simulink model "stepper_motor"  (R2015b)
settings: Solver=FixedStepDiscrete  StartTime=0.0  StopTime=0.25  FixedStep=Ts  RelTol=1e-3
undefined symbols (not defined in the file): DiscIntNeverNeededParam, Ts
settings Model: Creator=YogurtSuee  LastModifiedBy=YogurtSuee

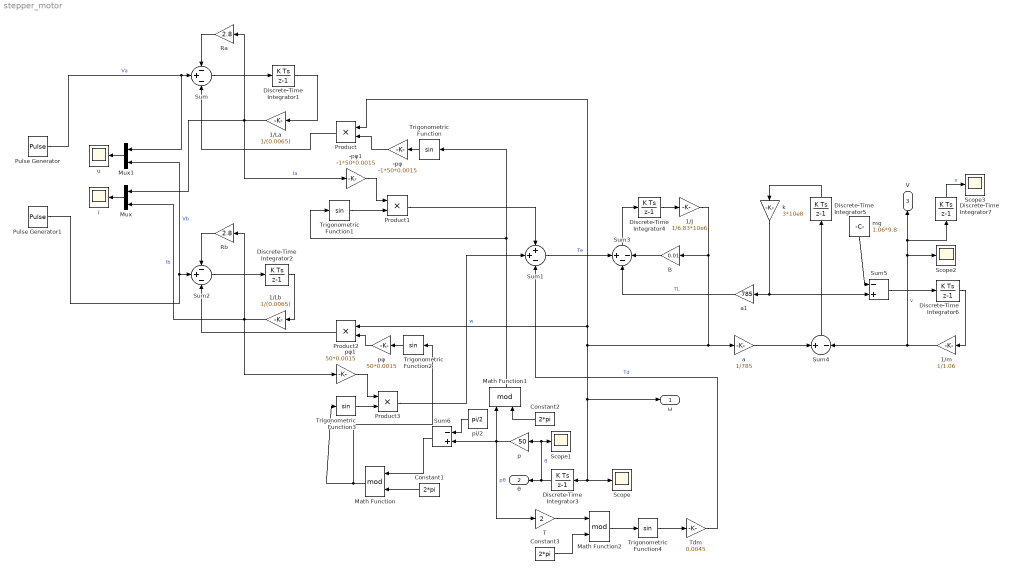
== system stepper_motor ==
  -pφ : Gain  Gain=-1*50*0.0015
  -pφ1 : Gain  Gain=-1*50*0.0015
  1/J : Gain  Gain=1/6.83*10e6
  1/La : Gain  Gain=1/(0.0065)
  1/Lb : Gain  Gain=1/(0.0065)
  1/m : Gain  Gain=1/1.06
  B : Gain  Gain=0.01
  Constant1 : Constant  Value=2*pi
  Constant2 : Constant  Value=2*pi
  Constant3 : Constant  Value=2*pi
  Discrete-Time Integrator{1..7} (7 alike) : DiscreteIntegrator  SampleTime=Ts  ICPrevOutput=DiscIntNeverNeededParam  ICPrevScaledInput=DiscIntNeverNeededParam
  Math Function : Math  Operator=mod  SaturateOnIntegerOverflow=on
  Math Function1 : Math  Operator=mod  SaturateOnIntegerOverflow=on
  Math Function2 : Math  Operator=mod  SaturateOnIntegerOverflow=on
  Mux : Mux  Inputs=2
  Mux1 : Mux  Inputs=2
  Product{,1..3} (4 alike) : Product
  Pulse Generator : DiscretePulseGenerator  PulseType=Time based  Amplitude=24  Period=0.02  PulseWidth=10  SampleTime=0.2
  Pulse Generator1 : DiscretePulseGenerator  PulseType=Time based  Amplitude=24  Period=0.02  PulseWidth=10  PhaseDelay=0.01  SampleTime=0.2
  Ra : Gain  Gain=2.8
  Rb : Gain  Gain=2.8
  Scope{,1..3} (4 alike) : Scope
  Sum : Sum  Inputs=-+-
  Sum1 : Sum  Inputs=++-
  Sum2 : Sum  Inputs=-+-
  Sum3 : Sum  Inputs=+--
  Sum4 : Sum  Inputs=+-
  Sum5 : Sum  Inputs=-+
  Sum6 : Sum  Inputs=-+
  T : Gain  Gain=2
  Tdm : Gain  Gain=0.0045
  Trigonometric Function{,1..2,4} (4 alike) : Trigonometry
  Trigonometric Function3 : Trigonometry  OutputSignalType=real
  a : Gain  Gain=1/785
  a1 : Gain  Gain=785
  i : Scope
  k : Gain  Gain=3*10e8
  mg : Constant  Value=1.06*9.8
  p : Gain  Gain=50
  pi/2 : Constant  Value=pi/2
  pφ : Gain  Gain=50*0.0015
  pφ1 : Gain  Gain=50*0.0015
  u : Scope
  ω : Outport
  θ : Outport  Port=2
  V : Outport  Port=3
  wires:
  Discrete-Time Integrator1/1 -> 1/La/1
  Sum/1 -> Discrete-Time Integrator1/1
  Ra/1 -> Sum/1
  1/La/1 -> -pφ1/1, Mux/1, Ra/1  "Ia"
  Product/1 -> Sum/3
  -pφ1/1 -> Product1/1
  Trigonometric Function1/1 -> Product1/2
  Product1/1 -> Sum1/1
  Discrete-Time Integrator2/1 -> 1/Lb/1
  Sum2/1 -> Discrete-Time Integrator2/1
  Rb/1 -> Sum2/1
  1/Lb/1 -> pφ1/1, Mux/2, Rb/1  "Ib"
  Product2/1 -> Sum2/3
  pφ1/1 -> Product3/1
  Trigonometric Function3/1 -> Product3/2
  Product3/1 -> Sum1/2
  Tdm/1 -> Sum1/3  "Td"
  1/J/1 -> ω/1, Discrete-Time Integrator3/1, Scope/1, Product2/1, Product/1, a/1, B/1  "w"
  Sum3/1 -> Discrete-Time Integrator4/1
  Discrete-Time Integrator4/1 -> 1/J/1
  a1/1 -> Sum3/2  "TL"
  k/1 -> Sum5/2, a1/1
  Discrete-Time Integrator5/1 -> k/1
  a/1 -> Sum4/1
  Sum4/1 -> Discrete-Time Integrator5/1
  mg/1 -> Sum5/1
  Sum5/1 -> Discrete-Time Integrator6/1
  Discrete-Time Integrator6/1 -> 1/m/1
  1/m/1 -> Scope2/1, Discrete-Time Integrator7/1, V/1, Sum4/2  "v"
  Discrete-Time Integrator3/1 -> Scope1/1, p/1, θ/1  "θ"
  p/1 -> Sum6/2, T/1, Math Function1/1  "pθ"
  pi/2/1 -> Sum6/1
  Discrete-Time Integrator7/1 -> Scope3/1  "x"
  Mux/1 -> i/1
  Mux1/1 -> u/1
  Trigonometric Function4/1 -> Tdm/1
  Constant1/1 -> Math Function/2
  Sum6/1 -> Math Function/1
  Math Function/1 -> Trigonometric Function3/1, Trigonometric Function2/1
  Constant2/1 -> Math Function1/2
  Math Function1/1 -> Trigonometric Function/1, Trigonometric Function1/1
  Constant3/1 -> Math Function2/2
  T/1 -> Math Function2/1
  Math Function2/1 -> Trigonometric Function4/1
  Sum1/1 -> Sum3/1  "Te"
  B/1 -> Sum3/3
  Trigonometric Function/1 -> -pφ/1
  -pφ/1 -> Product/2
  Trigonometric Function2/1 -> pφ/1
  pφ/1 -> Product2/2
  Pulse Generator/1 -> Mux1/1, Sum/2  "Va"
  Pulse Generator1/1 -> Mux1/2, Sum2/2  "Vb"
